simulink model "mg_test18"  (R2017b)
settings: Solver=VariableStepAuto  StartTime=0.0  StopTime=3  MaxStep=1e-4  RelTol=1e-3
values from neighbouring files (symbols this model uses):
  f = 50    [param_mgtest17.m]
  L = 0.15*Pbase/(2*pi*f)    (= 0.000459957785536)    [param_mgtest17.m]
  RL = 1.5e-3*Pbase    (= 0.001445)    [param_mgtest17.m]
  Ts_Power = 1/(fs*100)    (= 2.0202020202e-06)    [param_mgtest17.m]
libraries: powerlib x48, powerlib_meascontrol x15, simulink x8, re_lib x2, electricdrivelib x2, pePowerMeasurement x1
(part 1 of 2)
settings Model: Creator=vijay  LastModifiedBy=btp
settings SFSimCC: SimUseLocalCustomCode=on
settings RTWCC: RTWUseLocalCustomCode=on

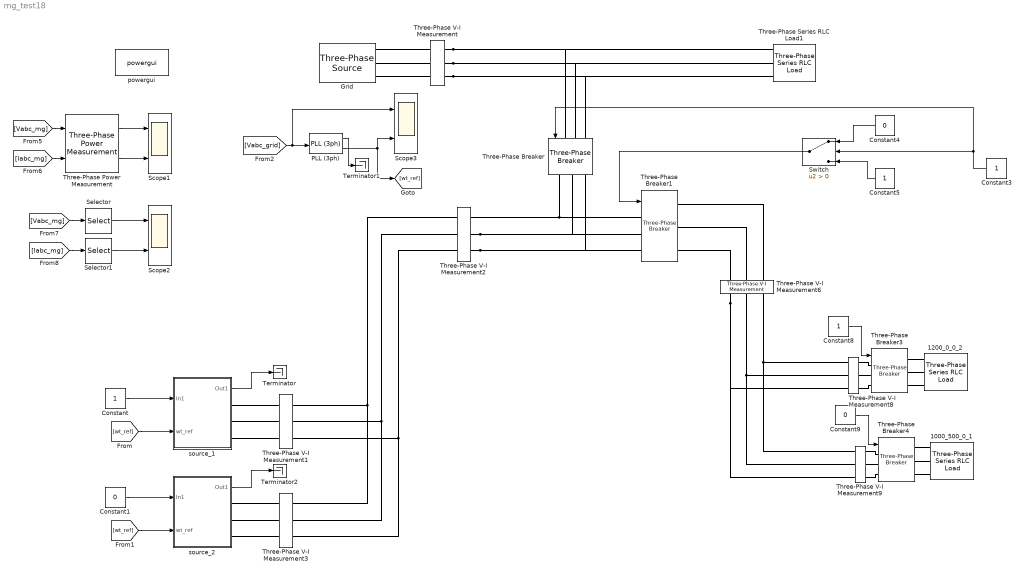
== system mg_test18 ==
  1000_500_0_1 : powerlib/Elements/Three-Phase Series RLC Load  LConnTagsString=A|B|C  Configuration=Y (grounded)  NominalVoltage=230  Vabc=[1e3 1e3 1e3]  Vabcp=[1e3 1e3 1e3]  NominalFrequency=f  UnbalancedPower=off  ActivePower=1e3  InductivePower=500  CapacitivePower=0  Pabc=[10e3 9e3 11e3]  QLabc=[100 90 110]  QCabc=[100 90 110]  Pabcp=[10e3 9e3 11e3]  QLabcp=[100 90 110]  QCabcp=[100 90 110]  Measurements=None  LoadType=constant Z
  1200_0_0_2 : powerlib/Elements/Three-Phase Series RLC Load  LConnTagsString=A|B|C  Configuration=Y (grounded)  NominalVoltage=230  Vabc=[1e3 1e3 1e3]  Vabcp=[1e3 1e3 1e3]  NominalFrequency=f  UnbalancedPower=off  ActivePower=1.2e3  InductivePower=0  CapacitivePower=0  Pabc=[10e3 9e3 11e3]  QLabc=[100 90 110]  QCabc=[100 90 110]  Pabcp=[10e3 9e3 11e3]  QLabcp=[100 90 110]  QCabcp=[100 90 110]  Measurements=None  LoadType=constant Z
  Constant{,3,5,8} (4 alike) : Constant
  Constant1 : Constant  Value=0
  Constant4 : Constant  Value=0
  Constant9 : Constant  Value=0
  Grid : powerlib/Electrical Sources/Three-Phase Source  InternalConnection=Yg  VoltagePhases=off  Voltage=230  PhaseAngle=0  Voltage_phases=[25e3 25e3 25e3]/sqrt(3)  PhaseAngles_phases=[0 -120 +120]  Frequency=f  NonIdealSource=on  SpecifyImpedance=off  Resistance=0.8929  Inductance=16.58e-3  ShortCircuitLevel=100e6  BaseVoltage=230  XRratio=7  BusType=swing  Pref=10e3  Qref=0  Prefabc=[10e3, 10e3, 10e3]  Qrefabc=[0, 0, 0]  Qmin=-inf  Qmax=inf
  PLL (3ph) : powerlib_meascontrol/PLL/PLL (3ph)  Fmin=45  Par_Init=[0, 60]  ParK=[180, 3200, 1]  TcD=1e-4  MaxRateChangeFreq=12  FilterCutOffFreq=25  Ts=0  AGC=on
  Scope1 : Scope  NumInputPorts=2
  Scope2 : Scope  NumInputPorts=2
  Scope3 : Scope  NumInputPorts=2
  Selector : Selector  InputPortWidth=3  IndexOptions=Index vector (dialog)  Indices=[1 ]  OutputSizes=1
  Selector1 : Selector  InputPortWidth=3  IndexOptions=Index vector (dialog)  Indices=[1 ]  OutputSizes=1
  Switch : Switch  Criteria=u2 > Threshold
  Terminator : Terminator
  Terminator1 : Terminator
  Terminator2 : Terminator
  Three-Phase Series RLC Load1 : powerlib/Elements/Three-Phase Series RLC Load  LConnTagsString=A|B|C  Configuration=Y (grounded)  NominalVoltage=230  Vabc=[1e3 1e3 1e3]  Vabcp=[1e3 1e3 1e3]  NominalFrequency=f  UnbalancedPower=off  ActivePower=10e3  InductivePower=0  CapacitivePower=0  Pabc=[10e3 9e3 11e3]  QLabc=[100 90 110]  QCabc=[100 90 110]  Pabcp=[10e3 9e3 11e3]  QLabcp=[100 90 110]  QCabcp=[100 90 110]  Measurements=None  LoadType=constant Z
  Three-Phase V-I Measurement : powerlib/Measurements/Three-Phase V-I Measurement  VoltageMeasurement=phase-to-phase  SetLabelV=on  LabelV=Vabc_grid  Vpu=off  VpuLL=off  CurrentMeasurement=yes  SetLabelI=on  LabelI=Iabc_grid  Ipu=off  Pbase=100e6  Vbase=500e3  OutputType=Complex  PhasorSimulation=off  PSBequivalent=0
  Three-Phase V-I Measurement1 : powerlib/Measurements/Three-Phase V-I Measurement  VoltageMeasurement=phase-to-ground  SetLabelV=on  LabelV=Vabc_s1  Vpu=off  VpuLL=off  CurrentMeasurement=yes  SetLabelI=on  LabelI=Iabc_s1  Ipu=off  Pbase=100e6  Vbase=500e3  OutputType=Complex  PhasorSimulation=off  PSBequivalent=0
  Three-Phase V-I Measurement2 : powerlib/Measurements/Three-Phase V-I Measurement  VoltageMeasurement=phase-to-ground  SetLabelV=on  LabelV=Vabc_mg  Vpu=off  VpuLL=off  CurrentMeasurement=yes  SetLabelI=on  LabelI=Iabc_mg  Ipu=off  Pbase=100e6  Vbase=500e3  OutputType=Complex  PhasorSimulation=off  PSBequivalent=0
  Three-Phase V-I Measurement3 : powerlib/Measurements/Three-Phase V-I Measurement  VoltageMeasurement=phase-to-ground  SetLabelV=on  LabelV=Vabc_s2  Vpu=off  VpuLL=off  CurrentMeasurement=yes  SetLabelI=on  LabelI=Iabc_s2  Ipu=off  Pbase=100e6  Vbase=500e3  OutputType=Complex  PhasorSimulation=off  PSBequivalent=0
  Three-Phase V-I Measurement6 : powerlib/Measurements/Three-Phase V-I Measurement  VoltageMeasurement=phase-to-ground  SetLabelV=on  LabelV=Vabc_mgl  Vpu=off  VpuLL=off  CurrentMeasurement=yes  SetLabelI=on  LabelI=Iabc_mgl  Ipu=off  Pbase=100e6  Vbase=500e3  OutputType=Complex  PhasorSimulation=off  PSBequivalent=0
  Three-Phase V-I Measurement8 : powerlib/Measurements/Three-Phase V-I Measurement  VoltageMeasurement=phase-to-ground  SetLabelV=on  LabelV=Vabc_l2  Vpu=off  VpuLL=off  CurrentMeasurement=yes  SetLabelI=on  LabelI=Iabc_l2  Ipu=off  Pbase=100e6  Vbase=500e3  OutputType=Complex  PhasorSimulation=off  PSBequivalent=0
  Three-Phase V-I Measurement9 : powerlib/Measurements/Three-Phase V-I Measurement  VoltageMeasurement=phase-to-ground  SetLabelV=on  LabelV=Vabc_l3  Vpu=off  VpuLL=off  CurrentMeasurement=yes  SetLabelI=on  LabelI=Iabc_l3  Ipu=off  Pbase=100e6  Vbase=500e3  OutputType=Complex  PhasorSimulation=off  PSBequivalent=0
  Three-Phase Breaker{,1,3..4} (4 alike) : powerlib/Elements/Three-Phase Breaker  InitialState=open  SwitchA=on  SwitchB=on  SwitchC=on  SwitchTimes="[1/60  5/60]"  External=on  BreakerResistance=0.01  SnubberResistance=1e6  SnubberCapacitance=inf  Measurements=None
  Three-Phase Power Measurement : pePowerMeasurement/Three-Phase Power Measurement  OverrideUsingVariant=Continuous  F=f  K=[0 1 2 3]  Seq=Positive  Ts=0
  powergui : powerlib/powergui  Priority=1  SimulationMode=Continuous  SampleTime=Ts_Power  frequency=60  Iterations=50  frequencyindice=0  Pbase=100e6  ErrMax=1e-4  UnitsV=kV  UnitsW=MW  buscounter=0  FunctionMessages=off  echomessages=off  EnableUseOfTLC=off  CurrentSourceSwitches=off  DisableSnubberDevices=off  DisableRonSwitches=off  DisableVfSwitches=off  DisplayEquations=off  SolverType=Tustin/Backward Euler (TBE)  Interpol=off  ExternalGateDelay=off  methode=off  Ts=100  x0status=blocks  SPID=on  SwTol=0  HookPort=off  RestoreLinks=warning  ResistiveCurrentMeasurement=off  Frange=[0:2:500]  Ylog=off  Xlog=on  ShowGrid=off  save=off  variable=ZData  structure=0  ZoomFFT=off  StartTime=0.0  cycles=1  DisplayStyle=1  fundamental=60  FreqAxis=off  MaxFrequency=1000  frequencyindicesteady=1  RmsSteady=1  display=off
  source_1 : Subsystem
  source_2 : Subsystem
  wires:
  source_2/1(Out1) -> Terminator2/1
  [wt_ref] -> source_2/2(wt_ref)
  Constant1/1 -> source_2/1(In1)
  [Vabc_mg] -> Three-Phase Power Measurement/1
  Three-Phase Power Measurement/2 -> Scope1/2
  Three-Phase Power Measurement/1 -> Scope1/1
  [Iabc_mg] -> Three-Phase Power Measurement/2
  Selector1/1 -> Scope2/2
  Selector/1 -> Scope2/1
  Constant8/1 -> Three-Phase Breaker3/1
  [wt_ref] -> source_1/2(wt_ref)
  Constant3/1 -> Three-Phase Breaker/1, Switch/2
  [Vabc_mg] -> Selector/1
  PLL (3ph)/2 -> [wt_ref], Scope3/2
  PLL (3ph)/1 -> Terminator1/1
  Constant/1 -> source_1/1(In1)
  Constant5/1 -> Switch/3
  Switch/1 -> Three-Phase Breaker1/1
  source_1/1(Out1) -> Terminator/1
  [Vabc_grid] -> Scope3/1, PLL (3ph)/1
  Constant4/1 -> Switch/1
  [Iabc_mg] -> Selector1/1
  Constant9/1 -> Three-Phase Breaker4/1
  connections:
  Three-Phase V-I Measurement2/LConn3 -- Three-Phase V-I Measurement3/RConn3 -- Three-Phase V-I Measurement1/RConn3
  Three-Phase V-I Measurement/RConn2 -- Three-Phase Series RLC Load1/LConn2 -- Three-Phase Breaker/LConn2
  Three-Phase V-I Measurement2/LConn1 -- Three-Phase V-I Measurement3/RConn1 -- Three-Phase V-I Measurement1/RConn1
  Three-Phase V-I Measurement2/LConn2 -- Three-Phase V-I Measurement3/RConn2 -- Three-Phase V-I Measurement1/RConn2
  Three-Phase V-I Measurement/RConn3 -- Three-Phase Series RLC Load1/LConn3 -- Three-Phase Breaker/LConn3
  Three-Phase V-I Measurement6/RConn3 -- Three-Phase V-I Measurement9/LConn3 -- Three-Phase V-I Measurement8/LConn3
  Three-Phase V-I Measurement8/LConn2 -- Three-Phase V-I Measurement9/LConn2 -- Three-Phase V-I Measurement6/RConn2
  Three-Phase V-I Measurement2/RConn3 -- Three-Phase Breaker1/LConn3 -- Three-Phase Breaker/RConn3
  Three-Phase V-I Measurement8/LConn1 -- Three-Phase V-I Measurement9/LConn1 -- Three-Phase V-I Measurement6/RConn1
  Three-Phase Breaker1/LConn1 -- Three-Phase Breaker/RConn1 -- Three-Phase V-I Measurement2/RConn1
  Three-Phase V-I Measurement/RConn1 -- Three-Phase Series RLC Load1/LConn1 -- Three-Phase Breaker/LConn1
  Three-Phase V-I Measurement2/RConn2 -- Three-Phase Breaker1/LConn2 -- Three-Phase Breaker/RConn2
  source_2/RConn1 -- Three-Phase V-I Measurement3/LConn1
  Three-Phase Breaker3/RConn2 -- 1200_0_0_2/LConn2
  source_2/RConn2 -- Three-Phase V-I Measurement3/LConn2
  Three-Phase Breaker3/RConn1 -- 1200_0_0_2/LConn1
  source_2/RConn3 -- Three-Phase V-I Measurement3/LConn3
  Three-Phase V-I Measurement8/RConn1 -- Three-Phase Breaker3/LConn1
  Three-Phase V-I Measurement8/RConn3 -- Three-Phase Breaker3/LConn3
  Three-Phase V-I Measurement8/RConn2 -- Three-Phase Breaker3/LConn2
  Grid/RConn2 -- Three-Phase V-I Measurement/LConn2
  Three-Phase V-I Measurement9/RConn1 -- Three-Phase Breaker4/LConn1
  Grid/RConn3 -- Three-Phase V-I Measurement/LConn3
  Three-Phase Breaker4/RConn3 -- 1000_500_0_1/LConn3
  Three-Phase V-I Measurement1/LConn3 -- source_1/RConn3
  Three-Phase V-I Measurement1/LConn1 -- source_1/RConn1
  Grid/RConn1 -- Three-Phase V-I Measurement/LConn1
  Three-Phase V-I Measurement6/LConn2 -- Three-Phase Breaker1/RConn2
  Three-Phase V-I Measurement6/LConn3 -- Three-Phase Breaker1/RConn3
  Three-Phase Breaker4/RConn1 -- 1000_500_0_1/LConn1
  Three-Phase V-I Measurement9/RConn2 -- Three-Phase Breaker4/LConn2
  Three-Phase Breaker3/RConn3 -- 1200_0_0_2/LConn3
  Three-Phase V-I Measurement6/LConn1 -- Three-Phase Breaker1/RConn1
  Three-Phase V-I Measurement9/RConn3 -- Three-Phase Breaker4/LConn3
  Three-Phase V-I Measurement1/LConn2 -- source_1/RConn2
  Three-Phase Breaker4/RConn2 -- 1000_500_0_1/LConn2

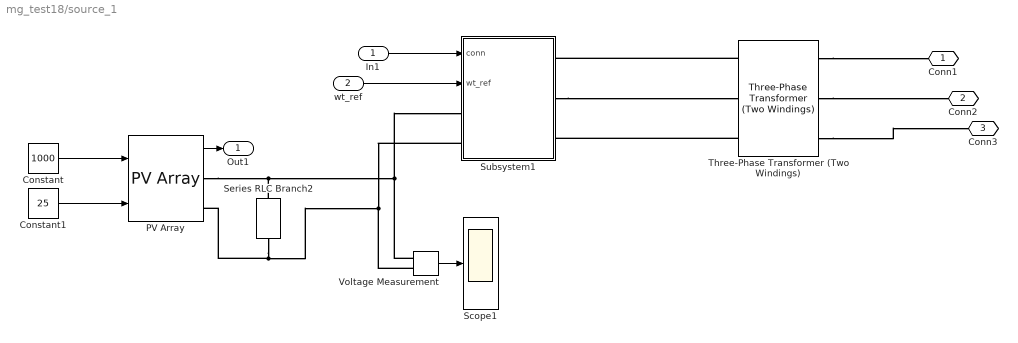
== system mg_test18/source_1 ==
  In1 : Inport
  wt_ref : Inport  Port=2
  Constant : Constant  Value=1000
  Constant1 : Constant  Value=25
  PV Array : re_lib/Solar/PV Array  Npar=6  Nser=2  PlotType=array @ 1000 W/m2 & specified temperatures  S_vec="[ 1000  500  100 ]"  Temp_C_vec="[ 45 25  ]"  ModuleName=Zytech Engineering Technology ZT190S  PlotWhenSelected=off  Pm=190.1592  Ncell=72  Voc=44.86  Isc=5.5  Vm=37.73  Im=5.04  beta_Voc_pc=-0.364  alpha_Isc_pc=0.102  beta_Voc=-0.16329  alpha_Isc=0.00561  IL=5.5086  I0=2.2516e-10  nI=1.0158  Rsh=179.2693  Rs=0.2794  BAL=off  Tc=1e-6  Tfilter=5e-5
  Scope1 : Scope
  Series RLC Branch2 : powerlib/Elements/Series RLC Branch  LConnTagsString=__new0  RConnTagsString=__new0  BranchType=C  Resistance=1  Inductance=100e-3  SetiL0=off  InitialCurrent=0  Capacitance=470e-6  Setx0=on  InitialVoltage=60  Measurements=None
  Subsystem1 : Subsystem
  Three-Phase Transformer (Two Windings) : powerlib/Elements/Three-Phase Transformer (Two Windings)  Winding1Connection=Yg  Winding2Connection=Yg  CoreType=Three single-phase transformers  SetSaturation=off  Hysteresis=off  DataFile='hysteresis'  SetInitialFlux=off  Measurements=None  UNITS=pu  NominalPower=[ 1.2e3 , 50 ]  Winding1=[ 34 , 0.002 , 0.08 ]  Winding2=[ 230 , 0.002 , 0.08 ]  Rm=500  Lm=500  L0=0.5  Saturation=[ 0,0 ; 0.0024,1.2 ; 1.0,1.52 ]  InitialFluxes=[ 0.8 , -0.8 , 0.7 ]  MoreParameters=off  BreakLoop=off  DataType=off  TransfoNumber=1
  Voltage Measurement : powerlib/Measurements/Voltage Measurement  PhasorSimulation=off  OutputType=Complex  PSBequivalent=0
  Conn1 : PMIOPort  Port=1  Side=Right
  Conn2 : PMIOPort  Port=2  Side=Right
  Conn3 : PMIOPort  Port=3  Side=Right
  Out1 : Outport
  wires:
  Constant1/1 -> PV Array/2
  PV Array/1 -> Out1/1
  Constant/1 -> PV Array/1
  Voltage Measurement/1 -> Scope1/1
  In1/1 -> Subsystem1/1(conn)
  wt_ref/1 -> Subsystem1/2(wt_ref)
  connections:
  Subsystem1/RConn2 -- Three-Phase Transformer (Two Windings)/LConn2
  Series RLC Branch2/LConn1 -- Subsystem1/LConn1 -- Voltage Measurement/LConn1 -- PV Array/RConn1
  Three-Phase Transformer (Two Windings)/LConn3 -- Subsystem1/RConn3
  Three-Phase Transformer (Two Windings)/LConn1 -- Subsystem1/RConn1
  Voltage Measurement/LConn2 -- PV Array/RConn2 -- Series RLC Branch2/RConn1 -- Subsystem1/LConn2
  Three-Phase Transformer (Two Windings)/RConn3 -- Conn3/RConn1
  Three-Phase Transformer (Two Windings)/RConn2 -- Conn2/RConn1
  Three-Phase Transformer (Two Windings)/RConn1 -- Conn1/RConn1

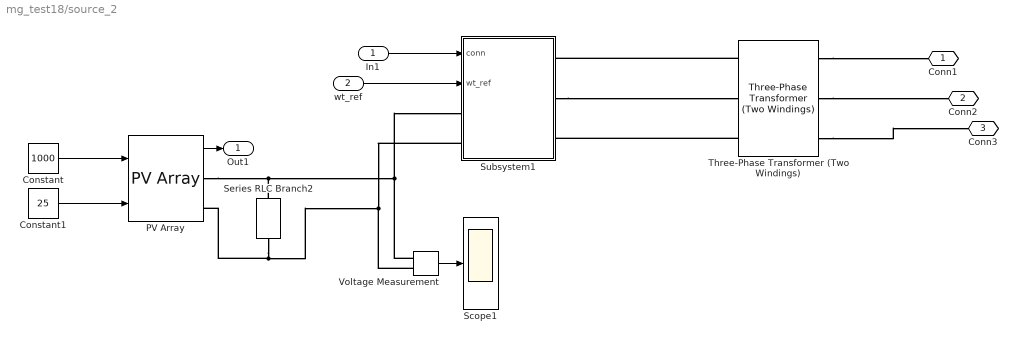
== system mg_test18/source_2 ==
  In1 : Inport
  wt_ref : Inport  Port=2
  Constant : Constant  Value=1000
  Constant1 : Constant  Value=25
  PV Array : re_lib/Solar/PV Array  Npar=6  Nser=2  PlotType=array @ 1000 W/m2 & specified temperatures  S_vec="[ 1000  500  100 ]"  Temp_C_vec="[ 45 25  ]"  ModuleName=Zytech Engineering Technology ZT190S  PlotWhenSelected=off  Pm=190.1592  Ncell=72  Voc=44.86  Isc=5.5  Vm=37.73  Im=5.04  beta_Voc_pc=-0.364  alpha_Isc_pc=0.102  beta_Voc=-0.16329  alpha_Isc=0.00561  IL=5.5086  I0=2.2516e-10  nI=1.0158  Rsh=179.2693  Rs=0.2794  BAL=off  Tc=1e-6  Tfilter=5e-5
  Scope1 : Scope
  Series RLC Branch2 : powerlib/Elements/Series RLC Branch  LConnTagsString=__new0  RConnTagsString=__new0  BranchType=C  Resistance=1  Inductance=100e-3  SetiL0=off  InitialCurrent=0  Capacitance=470e-6  Setx0=on  InitialVoltage=60  Measurements=None
  Subsystem1 : Subsystem
  Three-Phase Transformer (Two Windings) : powerlib/Elements/Three-Phase Transformer (Two Windings)  Winding1Connection=Yg  Winding2Connection=Yg  CoreType=Three single-phase transformers  SetSaturation=off  Hysteresis=off  DataFile='hysteresis'  SetInitialFlux=off  Measurements=None  UNITS=pu  NominalPower=[ 1.2e3 , 50 ]  Winding1=[ 34 , 0.002 , 0.08 ]  Winding2=[ 230 , 0.002 , 0.08 ]  Rm=500  Lm=500  L0=0.5  Saturation=[ 0,0 ; 0.0024,1.2 ; 1.0,1.52 ]  InitialFluxes=[ 0.8 , -0.8 , 0.7 ]  MoreParameters=off  BreakLoop=off  DataType=off  TransfoNumber=1
  Voltage Measurement : powerlib/Measurements/Voltage Measurement  PhasorSimulation=off  OutputType=Complex  PSBequivalent=0
  Conn1 : PMIOPort  Port=1  Side=Right
  Conn2 : PMIOPort  Port=2  Side=Right
  Conn3 : PMIOPort  Port=3  Side=Right
  Out1 : Outport
  wires:
  Constant1/1 -> PV Array/2
  PV Array/1 -> Out1/1
  Constant/1 -> PV Array/1
  Voltage Measurement/1 -> Scope1/1
  In1/1 -> Subsystem1/1(conn)
  wt_ref/1 -> Subsystem1/2(wt_ref)
  connections:
  Subsystem1/RConn2 -- Three-Phase Transformer (Two Windings)/LConn2
  Series RLC Branch2/LConn1 -- Subsystem1/LConn1 -- Voltage Measurement/LConn1 -- PV Array/RConn1
  Three-Phase Transformer (Two Windings)/LConn3 -- Subsystem1/RConn3
  Three-Phase Transformer (Two Windings)/LConn1 -- Subsystem1/RConn1
  Voltage Measurement/LConn2 -- PV Array/RConn2 -- Series RLC Branch2/RConn1 -- Subsystem1/LConn2
  Three-Phase Transformer (Two Windings)/RConn3 -- Conn3/RConn1
  Three-Phase Transformer (Two Windings)/RConn2 -- Conn2/RConn1
  Three-Phase Transformer (Two Windings)/RConn1 -- Conn1/RConn1

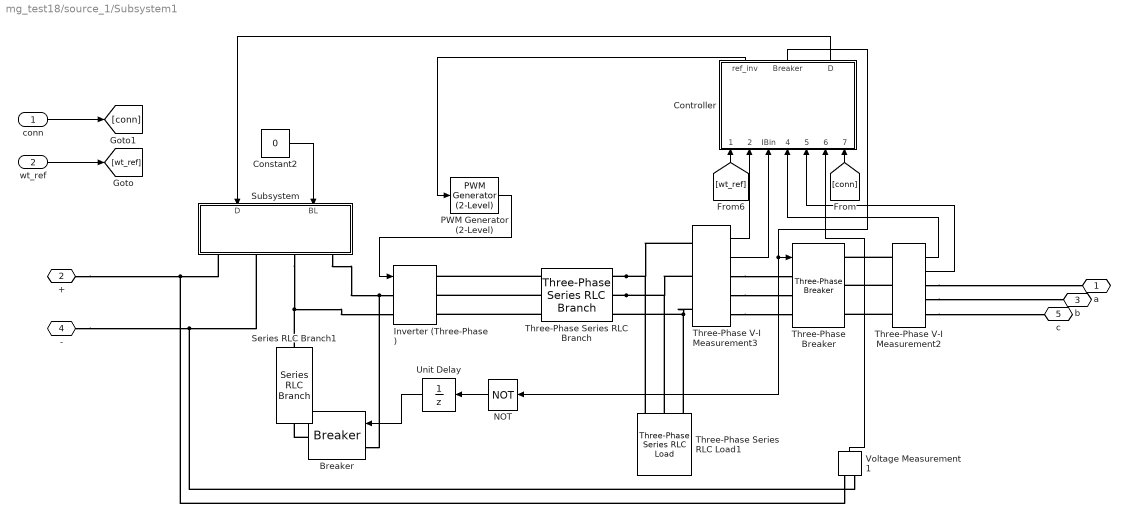
== system mg_test18/source_1/Subsystem1 ==
  conn : Inport
  wt_ref : Inport  Port=2
  Breaker : powerlib/Elements/Breaker  InitialState=0  SwitchingTimes="[1/60  5/60]"  External=on  BreakerResistance=0.01  SnubberResistance=1e6  SnubberCapacitance=inf  Measurements=None  MoreParameters=on  NoBreakLoop=off
      settings: SourceProductName=Simscape Power Systems
  Constant2 : Constant  Value=0
  "Controller " : Subsystem
  Inverter (Three-Phase) : electricdrivelib/Fundamental Drive Blocks/Inverter (Three-Phase)  OverrideUsingVariant=Detailed  detailLevel=Detailed  driveType=Field-oriented control  Ts=2e-6  SnubberResistance=1e6  SnubberCapacitance=inf  Device=IGBT / Diodes  Ron=1e-3  ForwardVoltages=[1.2,1.2]  GTOparameters=[1e-6,2e-6]  IGBTparameters=[1e-6,2e-6]  Measurements=All voltages and currents  converterType=Inverter  SourceFrequency=60  ReferenceFrame=Rotor  dqInductances=[8.5e-3,8.5e-3]  Inductance=8.5e-3  Ls=0  Resistance=0.2  Flux=0.175  Stator_sm=[2.01e-3,4.289e-4,4.477e-3,1.354e-3]  Stator_im=[14.85e-3,0.3027e-3]  Rotor=[9.295e-3,0.3027e-3]  Lm=10.46e-3  p=4
      settings: AttributesFormatString=%<BlockChoice>  SourceProductName=Simscape Power Systems  SourceProductBaseCode=PS
  NOT : Logic  Operator=NOT  IconShape=distinctive  AllPortsSameDT=off  OutDataTypeStr=boolean
  PWM Generator (2-Level) : powerlib_meascontrol/Pulse & Signal Generators/PWM Generator (2-Level)  ModulatorType=Three-phase bridge (6 pulses)  ModulatorMode=Unsynchronized  Fc=fs  Pc=90  nF=27  MinMax="[ -1  1 ]"  SamplingTechnique=Natural  ModulatingSignals=off  m=0.8  Freq=60  Phase=0  Ts=Ts_Power  ShowCarrierOutport=off
      settings: SourceProductName=Simscape Power Systems
  Series RLC Branch1 : powerlib/Elements/Series RLC Branch  LConnTagsString=__new0  RConnTagsString=__new0  BranchType=R  Resistance=1.92  Inductance=1e-3  SetiL0=off  InitialCurrent=0  Capacitance=1e-6  Setx0=off  InitialVoltage=0  Measurements=None
  Subsystem : Subsystem
  Three-Phase Series RLC Branch : powerlib/Elements/Three-Phase Series RLC Branch  LConnTagsString=A|B|C  RConnTagsString=A|B|C  BranchType=RL  Resistance=RL  Inductance=L  Capacitance=1e-6  Measurements=None
  Three-Phase Series RLC Load1 : powerlib/Elements/Three-Phase Series RLC Load  LConnTagsString=A|B|C  Configuration=Delta  NominalVoltage=Vbase  Vabc=[1e3 1e3 1e3]  Vabcp=[1e3 1e3 1e3]  NominalFrequency=f  UnbalancedPower=off  ActivePower=Pc  InductivePower=0  CapacitivePower=Qc  Pabc=[10e3 9e3 11e3]  QLabc=[100 90 110]  QCabc=[100 90 110]  Pabcp=[10e3 9e3 11e3]  QLabcp=[100 90 110]  QCabcp=[100 90 110]  Measurements=None  LoadType=constant Z
  Three-Phase V-I Measurement2 : powerlib/Measurements/Three-Phase V-I Measurement  VoltageMeasurement=phase-to-phase  SetLabelV=off  LabelV=v2  Vpu=off  VpuLL=off  CurrentMeasurement=yes  SetLabelI=off  LabelI=i2  Ipu=off  Pbase=100e6  Vbase=500e3  OutputType=Complex  PhasorSimulation=off  PSBequivalent=0
  Three-Phase V-I Measurement3 : powerlib/Measurements/Three-Phase V-I Measurement  VoltageMeasurement=phase-to-phase  SetLabelV=off  LabelV=v1  Vpu=off  VpuLL=off  CurrentMeasurement=yes  SetLabelI=off  LabelI=i1  Ipu=off  Pbase=100e6  Vbase=500e3  OutputType=Complex  PhasorSimulation=off  PSBequivalent=0
  Three-Phase Breaker : powerlib/Elements/Three-Phase Breaker  InitialState=open  SwitchA=on  SwitchB=on  SwitchC=on  SwitchTimes="[1/60  5/60]"  External=on  BreakerResistance=0.01  SnubberResistance=1e6  SnubberCapacitance=inf  Measurements=None
  Unit Delay : UnitDelay  InitialCondition=1  SampleTime=-1
  Voltage Measurement1 : powerlib/Measurements/Voltage Measurement  PhasorSimulation=off  OutputType=Complex  PSBequivalent=0
  a : PMIOPort  Port=1  Side=Right
  + : PMIOPort  Port=2  Side=Left
  b : PMIOPort  Port=3  Side=Right
  - : PMIOPort  Port=4  Side=Left
  c : PMIOPort  Port=5  Side=Right
  wires:
  PWM Generator (2-Level)/1 -> Inverter (Three-Phase)/1
  Constant2/1 -> Subsystem/2(BL)
  wt_ref/1 -> [wt_ref]
  conn/1 -> [conn]
  Three-Phase V-I Measurement3/1 -> "Controller "/2("VBin ")
  Three-Phase V-I Measurement3/2 -> "Controller "/3(IBin)
  Three-Phase V-I Measurement2/1 -> "Controller "/4(VBout)
  Three-Phase V-I Measurement2/2 -> "Controller "/5(IBout)
  Voltage Measurement1/1 -> "Controller "/6(In_DC)
  [conn] -> "Controller "/7(connect_o)
  [wt_ref] -> "Controller "/1(wt_ref)
  "Controller "/1(ref_inv) -> PWM Generator (2-Level)/1
  "Controller "/2("Breaker ") -> NOT/1, Three-Phase Breaker/1
  "Controller "/3("D ") -> Subsystem/1(D)
  NOT/1 -> Unit Delay/1
  Unit Delay/1 -> Breaker/1
  connections:
  Three-Phase V-I Measurement2/LConn2 -- Three-Phase Breaker/RConn2
  Voltage Measurement1/LConn1 -- +/RConn1 -- Subsystem/RConn1
  Voltage Measurement1/LConn2 -- Subsystem/RConn2 -- -/RConn1
  Three-Phase V-I Measurement3/RConn1 -- Three-Phase Breaker/LConn1
  Three-Phase V-I Measurement3/RConn3 -- Three-Phase Breaker/LConn3
  Subsystem/RConn4 -- Breaker/LConn1 -- Inverter (Three-Phase)/LConn1
  Three-Phase V-I Measurement2/LConn1 -- Three-Phase Breaker/RConn1
  Three-Phase V-I Measurement2/LConn3 -- Three-Phase Breaker/RConn3
  Subsystem/RConn3 -- Series RLC Branch1/LConn1 -- Inverter (Three-Phase)/LConn2
  Three-Phase V-I Measurement3/RConn2 -- Three-Phase Breaker/LConn2
  Three-Phase V-I Measurement2/RConn1 -- a/RConn1
  Three-Phase V-I Measurement2/RConn3 -- c/RConn1
  Three-Phase V-I Measurement2/RConn2 -- b/RConn1
  Three-Phase V-I Measurement3/LConn3 -- Three-Phase Series RLC Branch/RConn3 -- Three-Phase Series RLC Load1/LConn3
  Three-Phase Series RLC Branch/RConn1 -- Three-Phase V-I Measurement3/LConn1 -- Three-Phase Series RLC Load1/LConn1
  Three-Phase Series RLC Branch/RConn2 -- Three-Phase V-I Measurement3/LConn2 -- Three-Phase Series RLC Load1/LConn2
  Three-Phase Series RLC Branch/LConn3 -- Inverter (Three-Phase)/RConn3
  Three-Phase Series RLC Branch/LConn2 -- Inverter (Three-Phase)/RConn2
  Three-Phase Series RLC Branch/LConn1 -- Inverter (Three-Phase)/RConn1
  Breaker/RConn1 -- Series RLC Branch1/RConn1

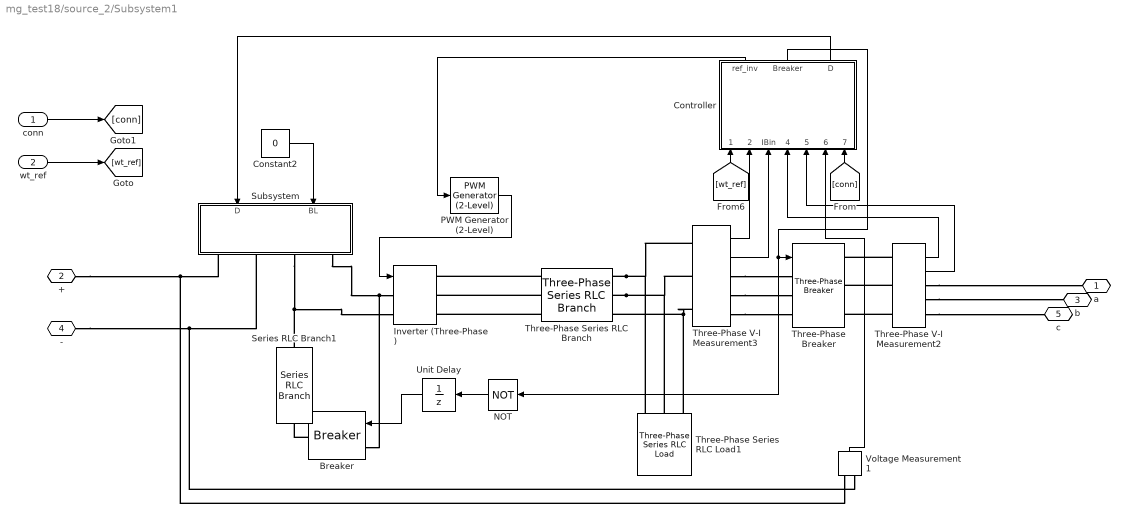
== system mg_test18/source_2/Subsystem1 ==
  conn : Inport
  wt_ref : Inport  Port=2
  Breaker : powerlib/Elements/Breaker  InitialState=0  SwitchingTimes="[1/60  5/60]"  External=on  BreakerResistance=0.01  SnubberResistance=1e6  SnubberCapacitance=inf  Measurements=None  MoreParameters=on  NoBreakLoop=off
      settings: SourceProductName=Simscape Power Systems
  Constant2 : Constant  Value=0
  "Controller " : Subsystem
  Inverter (Three-Phase) : electricdrivelib/Fundamental Drive Blocks/Inverter (Three-Phase)  OverrideUsingVariant=Detailed  detailLevel=Detailed  driveType=Field-oriented control  Ts=2e-6  SnubberResistance=1e6  SnubberCapacitance=inf  Device=IGBT / Diodes  Ron=1e-3  ForwardVoltages=[1.2,1.2]  GTOparameters=[1e-6,2e-6]  IGBTparameters=[1e-6,2e-6]  Measurements=All voltages and currents  converterType=Inverter  SourceFrequency=60  ReferenceFrame=Rotor  dqInductances=[8.5e-3,8.5e-3]  Inductance=8.5e-3  Ls=0  Resistance=0.2  Flux=0.175  Stator_sm=[2.01e-3,4.289e-4,4.477e-3,1.354e-3]  Stator_im=[14.85e-3,0.3027e-3]  Rotor=[9.295e-3,0.3027e-3]  Lm=10.46e-3  p=4
      settings: AttributesFormatString=%<BlockChoice>  SourceProductName=Simscape Power Systems  SourceProductBaseCode=PS
  NOT : Logic  Operator=NOT  IconShape=distinctive  AllPortsSameDT=off  OutDataTypeStr=boolean
  PWM Generator (2-Level) : powerlib_meascontrol/Pulse & Signal Generators/PWM Generator (2-Level)  ModulatorType=Three-phase bridge (6 pulses)  ModulatorMode=Unsynchronized  Fc=fs  Pc=90  nF=27  MinMax="[ -1  1 ]"  SamplingTechnique=Natural  ModulatingSignals=off  m=0.8  Freq=60  Phase=0  Ts=Ts_Power  ShowCarrierOutport=off
      settings: SourceProductName=Simscape Power Systems
  Series RLC Branch1 : powerlib/Elements/Series RLC Branch  LConnTagsString=__new0  RConnTagsString=__new0  BranchType=R  Resistance=1.92  Inductance=1e-3  SetiL0=off  InitialCurrent=0  Capacitance=1e-6  Setx0=off  InitialVoltage=0  Measurements=None
  Subsystem : Subsystem
  Three-Phase Series RLC Branch : powerlib/Elements/Three-Phase Series RLC Branch  LConnTagsString=A|B|C  RConnTagsString=A|B|C  BranchType=RL  Resistance=RL  Inductance=L  Capacitance=1e-6  Measurements=None
  Three-Phase Series RLC Load1 : powerlib/Elements/Three-Phase Series RLC Load  LConnTagsString=A|B|C  Configuration=Delta  NominalVoltage=Vbase  Vabc=[1e3 1e3 1e3]  Vabcp=[1e3 1e3 1e3]  NominalFrequency=f  UnbalancedPower=off  ActivePower=Pc  InductivePower=0  CapacitivePower=Qc  Pabc=[10e3 9e3 11e3]  QLabc=[100 90 110]  QCabc=[100 90 110]  Pabcp=[10e3 9e3 11e3]  QLabcp=[100 90 110]  QCabcp=[100 90 110]  Measurements=None  LoadType=constant Z
  Three-Phase V-I Measurement2 : powerlib/Measurements/Three-Phase V-I Measurement  VoltageMeasurement=phase-to-phase  SetLabelV=off  LabelV=v2  Vpu=off  VpuLL=off  CurrentMeasurement=yes  SetLabelI=off  LabelI=i2  Ipu=off  Pbase=100e6  Vbase=500e3  OutputType=Complex  PhasorSimulation=off  PSBequivalent=0
  Three-Phase V-I Measurement3 : powerlib/Measurements/Three-Phase V-I Measurement  VoltageMeasurement=phase-to-phase  SetLabelV=off  LabelV=v1  Vpu=off  VpuLL=off  CurrentMeasurement=yes  SetLabelI=off  LabelI=i1  Ipu=off  Pbase=100e6  Vbase=500e3  OutputType=Complex  PhasorSimulation=off  PSBequivalent=0
  Three-Phase Breaker : powerlib/Elements/Three-Phase Breaker  InitialState=open  SwitchA=on  SwitchB=on  SwitchC=on  SwitchTimes="[1/60  5/60]"  External=on  BreakerResistance=0.01  SnubberResistance=1e6  SnubberCapacitance=inf  Measurements=None
  Unit Delay : UnitDelay  InitialCondition=1  SampleTime=-1
  Voltage Measurement1 : powerlib/Measurements/Voltage Measurement  PhasorSimulation=off  OutputType=Complex  PSBequivalent=0
  a : PMIOPort  Port=1  Side=Right
  + : PMIOPort  Port=2  Side=Left
  b : PMIOPort  Port=3  Side=Right
  - : PMIOPort  Port=4  Side=Left
  c : PMIOPort  Port=5  Side=Right
  wires:
  PWM Generator (2-Level)/1 -> Inverter (Three-Phase)/1
  Constant2/1 -> Subsystem/2(BL)
  wt_ref/1 -> [wt_ref]
  conn/1 -> [conn]
  Three-Phase V-I Measurement3/1 -> "Controller "/2("VBin ")
  Three-Phase V-I Measurement3/2 -> "Controller "/3(IBin)
  Three-Phase V-I Measurement2/1 -> "Controller "/4(VBout)
  Three-Phase V-I Measurement2/2 -> "Controller "/5(IBout)
  Voltage Measurement1/1 -> "Controller "/6(In_DC)
  [conn] -> "Controller "/7(connect_o)
  [wt_ref] -> "Controller "/1(wt_ref)
  "Controller "/1(ref_inv) -> PWM Generator (2-Level)/1
  "Controller "/2("Breaker ") -> NOT/1, Three-Phase Breaker/1
  "Controller "/3("D ") -> Subsystem/1(D)
  NOT/1 -> Unit Delay/1
  Unit Delay/1 -> Breaker/1
  connections:
  Three-Phase V-I Measurement2/LConn2 -- Three-Phase Breaker/RConn2
  Voltage Measurement1/LConn1 -- +/RConn1 -- Subsystem/RConn1
  Voltage Measurement1/LConn2 -- Subsystem/RConn2 -- -/RConn1
  Three-Phase V-I Measurement3/RConn1 -- Three-Phase Breaker/LConn1
  Three-Phase V-I Measurement3/RConn3 -- Three-Phase Breaker/LConn3
  Subsystem/RConn4 -- Inverter (Three-Phase)/LConn1 -- Breaker/LConn1
  Three-Phase V-I Measurement2/LConn1 -- Three-Phase Breaker/RConn1
  Three-Phase V-I Measurement2/LConn3 -- Three-Phase Breaker/RConn3
  Subsystem/RConn3 -- Inverter (Three-Phase)/LConn2 -- Series RLC Branch1/LConn1
  Three-Phase V-I Measurement3/RConn2 -- Three-Phase Breaker/LConn2
  Three-Phase V-I Measurement2/RConn1 -- a/RConn1
  Three-Phase V-I Measurement2/RConn3 -- c/RConn1
  Three-Phase V-I Measurement2/RConn2 -- b/RConn1
  Three-Phase V-I Measurement3/LConn3 -- Three-Phase Series RLC Branch/RConn3 -- Three-Phase Series RLC Load1/LConn3
  Three-Phase Series RLC Branch/RConn1 -- Three-Phase V-I Measurement3/LConn1 -- Three-Phase Series RLC Load1/LConn1
  Three-Phase Series RLC Branch/RConn2 -- Three-Phase V-I Measurement3/LConn2 -- Three-Phase Series RLC Load1/LConn2
  Three-Phase Series RLC Branch/LConn3 -- Inverter (Three-Phase)/RConn3
  Three-Phase Series RLC Branch/LConn2 -- Inverter (Three-Phase)/RConn2
  Three-Phase Series RLC Branch/LConn1 -- Inverter (Three-Phase)/RConn1
  Breaker/RConn1 -- Series RLC Branch1/RConn1

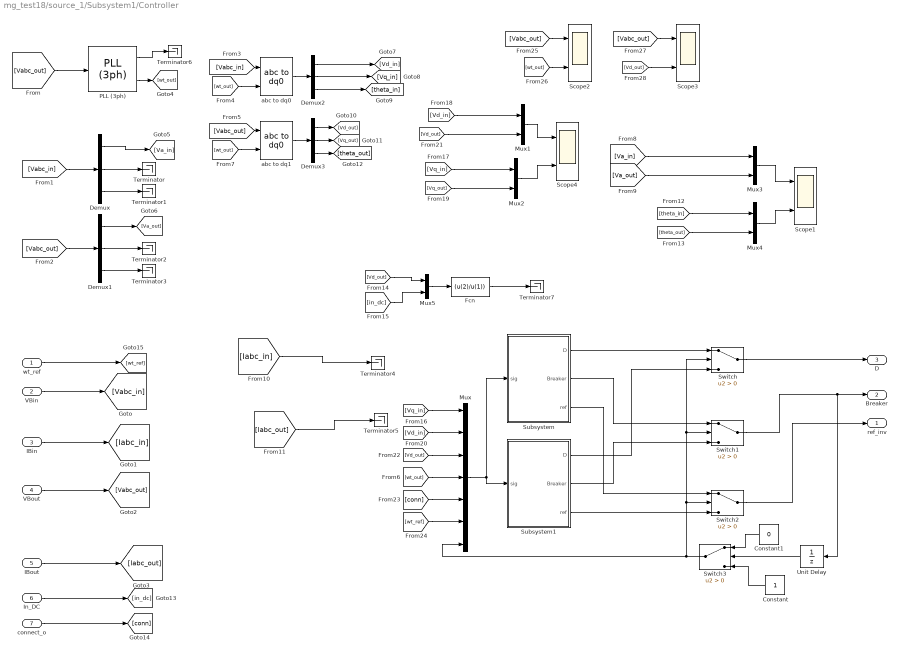
== system mg_test18/source_1/Subsystem1/Controller  ==
  wt_ref : Inport
  "VBin " : Inport  Port=2
  IBin : Inport  Port=3
  VBout : Inport  Port=4
  IBout : Inport  Port=5
  In_DC : Inport  Port=6
  connect_o : Inport  Port=7
  Constant : Constant
  Constant1 : Constant  Value=0
  Demux{,1..3} (4 alike) : Demux  Outputs=3
  Fcn : Fcn  Expr=(u(2)/u(1))
  Mux : Mux  Inputs=7
  Mux{1..5} (5 alike) : Mux  Inputs=2
  PLL (3ph) : powerlib_meascontrol/PLL/PLL (3ph)  Fmin=45  Par_Init=[0, f]  ParK=[180, 3200, 1]  TcD=1e-4  MaxRateChangeFreq=12  FilterCutOffFreq=25  Ts=Ts_Power  AGC=on
  Scope{1..4} (4 alike) : Scope  NumInputPorts=2
  Subsystem : Subsystem
  Subsystem1 : Subsystem
  Switch{,1..3} (4 alike) : Switch  Criteria=u2 > Threshold
  Terminator{,1..7} (8 alike) : Terminator
  Unit Delay : UnitDelay  SampleTime=Ts_Power
  abc to dq0 : powerlib_meascontrol/Transformations/abc to dq0  Alignment=90 degrees behind phase A axis
  abc to dq1 : powerlib_meascontrol/Transformations/abc to dq0  Alignment=90 degrees behind phase A axis
  ref_inv : Outport
  "Breaker " : Outport  Port=2
  "D " : Outport  Port=3
  wires:
  [Vd_out] -> Scope3/2
  [Vq_out] -> Mux2/2
  [wt_ref] -> Mux/6
  abc to dq1/1 -> Demux3/1
  [wt_out] -> Scope2/2
  [Vabc_out] -> Scope2/1
  [Iabc_out] -> Terminator5/1
  "VBin "/1 -> [Vabc_in]
  abc to dq0/1 -> Demux2/1
  Subsystem1/1(D) -> Switch/3
  [Vq_in] -> Mux/1
  Subsystem/2(Breaker) -> Switch1/1
  [Vq_in] -> Mux2/1
  [wt_out] -> abc to dq1/2
  PLL (3ph)/1 -> Terminator6/1
  In_DC/1 -> [in_dc]
  Switch1/1 -> Unit Delay/1, "Breaker "/1
  [conn] -> Mux/5
  Demux3/2 -> [Vq_out]
  [Vd_in] -> Mux/2
  Demux/2 -> Terminator/1
  Mux5/1 -> Fcn/1
  Switch2/1 -> ref_inv/1
  Fcn/1 -> Terminator7/1
  Subsystem/1(D) -> Switch/1
  [wt_out] -> Mux/4
  [Vd_out] -> Mux5/1
  Switch/1 -> "D "/1
  Mux/1 -> Subsystem/1(sig), Subsystem1/1(sig)
  [wt_out] -> abc to dq0/2
  [in_dc] -> Mux5/2
  [theta_out] -> Mux4/2
  [Vd_in] -> Mux1/1
  Mux2/1 -> Scope4/2
  [theta_in] -> Mux4/1
  wt_ref/1 -> [wt_ref]
  Mux4/1 -> Scope1/2
  Demux3/1 -> [Vd_out]
  Demux/1 -> [Va_in]
  connect_o/1 -> [conn]
  Mux1/1 -> Scope4/1
  Subsystem1/2(Breaker) -> Switch1/3
  [Vabc_in] -> abc to dq0/1
  [Vd_out] -> Mux1/2
  Subsystem/3(ref) -> Switch2/1
  Demux1/3 -> Terminator3/1
  [Va_in] -> Mux3/1
  Demux1/2 -> Terminator2/1
  [Iabc_in] -> Terminator4/1
  Demux/3 -> Terminator1/1
  [Vabc_out] -> PLL (3ph)/1
  [Vd_out] -> Mux/3
  [Vabc_out] -> abc to dq1/1
  [Va_out] -> Mux3/2
  Mux3/1 -> Scope1/1
  VBout/1 -> [Vabc_out]
  [Vabc_out] -> Demux1/1
  [Vabc_in] -> Demux/1
  PLL (3ph)/2 -> [wt_out]
  Subsystem1/3(ref) -> Switch2/3
  IBout/1 -> [Iabc_out]
  [Vabc_out] -> Scope3/1
  Demux3/3 -> [theta_out]
  IBin/1 -> [Iabc_in]
  Demux1/1 -> [Va_out]
  Demux2/3 -> [theta_in]
  Demux2/2 -> [Vq_in]
  Demux2/1 -> [Vd_in]
  Switch3/1 -> Switch/2, Switch1/2, Switch2/2, Mux/7
  Unit Delay/1 -> Switch3/2
  Constant/1 -> Switch3/3
  Constant1/1 -> Switch3/1

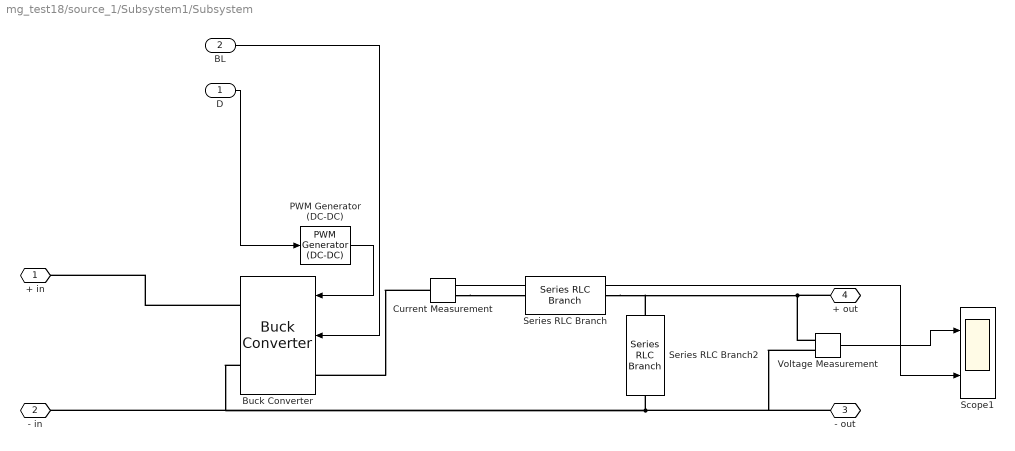
== system mg_test18/source_1/Subsystem1/Subsystem ==
  D : Inport
  BL : Inport  Port=2
  Buck Converter : powerlib/Power Electronics/Buck Converter  ModelType=Switching devices  Ron=1e-3  Rs=1e6  Cs=inf  Vforward=[0,0]  Ron_Diode=1e-3  Rs_Diode=1e6  Cs_Diode=inf  Vf_Diode=1e-3  Rs_CurrentSource=inf
      settings: SourceProductName=Simscape Power Systems  SourceProductBaseCode=PS
  Current Measurement : powerlib/Measurements/Current Measurement  PhasorSimulation=off  OutputType=Complex  PSBequivalent=0
  PWM Generator (DC-DC) : powerlib_meascontrol/Pulse & Signal Generators/PWM Generator (DC-DC)  Fsw=20000  Ts=0
  Scope1 : Scope  NumInputPorts=2
  Series RLC Branch : powerlib/Elements/Series RLC Branch  LConnTagsString=__new0  RConnTagsString=__new0  BranchType=L  Resistance=1  Inductance=96e-6  SetiL0=off  InitialCurrent=0  Capacitance=1e-6  Setx0=off  InitialVoltage=0  Measurements=None
  Series RLC Branch2 : powerlib/Elements/Series RLC Branch  LConnTagsString=__new0  RConnTagsString=__new0  BranchType=C  Resistance=1  Inductance=100e-3  SetiL0=off  InitialCurrent=0  Capacitance=470e-6  Setx0=on  InitialVoltage=0  Measurements=None
  Voltage Measurement : powerlib/Measurements/Voltage Measurement  PhasorSimulation=off  OutputType=Complex  PSBequivalent=0
  + in : PMIOPort  Port=1  Side=Right
  "- in " : PMIOPort  Port=2  Side=Right
  - out : PMIOPort  Port=3  Side=Right
  "+ out " : PMIOPort  Port=4  Side=Right
  wires:
  PWM Generator (DC-DC)/1 -> Buck Converter/1
  D/1 -> PWM Generator (DC-DC)/1
  Voltage Measurement/1 -> Scope1/1
  Current Measurement/1 -> Scope1/2
  BL/1 -> Buck Converter/2
  connections:
  Voltage Measurement/LConn1 -- Series RLC Branch/RConn1 -- Series RLC Branch2/LConn1 -- "+ out "/RConn1
  Series RLC Branch2/RConn1 -- - out/RConn1 -- Voltage Measurement/LConn2 -- "- in "/RConn1 -- Buck Converter/RConn2
  Current Measurement/RConn1 -- Series RLC Branch/LConn1
  Current Measurement/LConn1 -- Buck Converter/LConn1
  Buck Converter/RConn1 -- + in/RConn1

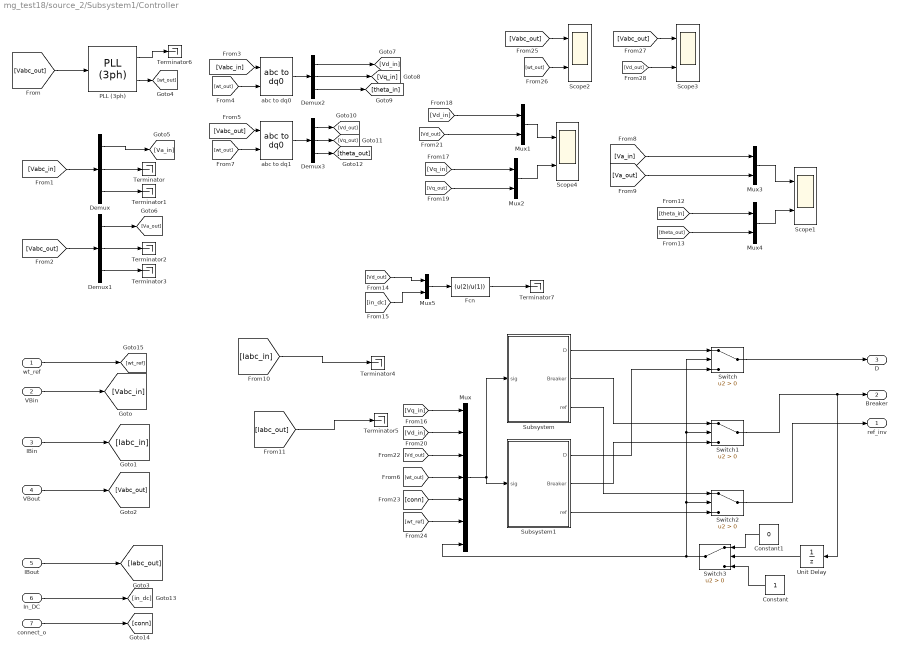
== system mg_test18/source_2/Subsystem1/Controller  ==
  wt_ref : Inport
  "VBin " : Inport  Port=2
  IBin : Inport  Port=3
  VBout : Inport  Port=4
  IBout : Inport  Port=5
  In_DC : Inport  Port=6
  connect_o : Inport  Port=7
  Constant : Constant
  Constant1 : Constant  Value=0
  Demux{,1..3} (4 alike) : Demux  Outputs=3
  Fcn : Fcn  Expr=(u(2)/u(1))
  Mux : Mux  Inputs=7
  Mux{1..5} (5 alike) : Mux  Inputs=2
  PLL (3ph) : powerlib_meascontrol/PLL/PLL (3ph)  Fmin=45  Par_Init=[0, f]  ParK=[180, 3200, 1]  TcD=1e-4  MaxRateChangeFreq=12  FilterCutOffFreq=25  Ts=Ts_Power  AGC=on
  Scope{1..4} (4 alike) : Scope  NumInputPorts=2
  Subsystem : Subsystem
  Subsystem1 : Subsystem
  Switch{,1..3} (4 alike) : Switch  Criteria=u2 > Threshold
  Terminator{,1..7} (8 alike) : Terminator
  Unit Delay : UnitDelay  SampleTime=Ts_Power
  abc to dq0 : powerlib_meascontrol/Transformations/abc to dq0  Alignment=90 degrees behind phase A axis
  abc to dq1 : powerlib_meascontrol/Transformations/abc to dq0  Alignment=90 degrees behind phase A axis
  ref_inv : Outport
  "Breaker " : Outport  Port=2
  "D " : Outport  Port=3
  wires:
  [Vd_out] -> Scope3/2
  [Vq_out] -> Mux2/2
  [wt_ref] -> Mux/6
  abc to dq1/1 -> Demux3/1
  [wt_out] -> Scope2/2
  [Vabc_out] -> Scope2/1
  [Iabc_out] -> Terminator5/1
  "VBin "/1 -> [Vabc_in]
  abc to dq0/1 -> Demux2/1
  Subsystem1/1(D) -> Switch/3
  [Vq_in] -> Mux/1
  Subsystem/2(Breaker) -> Switch1/1
  [Vq_in] -> Mux2/1
  [wt_out] -> abc to dq1/2
  PLL (3ph)/1 -> Terminator6/1
  In_DC/1 -> [in_dc]
  Switch1/1 -> Unit Delay/1, "Breaker "/1
  [conn] -> Mux/5
  Demux3/2 -> [Vq_out]
  [Vd_in] -> Mux/2
  Demux/2 -> Terminator/1
  Mux5/1 -> Fcn/1
  Switch2/1 -> ref_inv/1
  Fcn/1 -> Terminator7/1
  Subsystem/1(D) -> Switch/1
  [wt_out] -> Mux/4
  [Vd_out] -> Mux5/1
  Switch/1 -> "D "/1
  Mux/1 -> Subsystem/1(sig), Subsystem1/1(sig)
  [wt_out] -> abc to dq0/2
  [in_dc] -> Mux5/2
  [theta_out] -> Mux4/2
  [Vd_in] -> Mux1/1
  Mux2/1 -> Scope4/2
  [theta_in] -> Mux4/1
  wt_ref/1 -> [wt_ref]
  Mux4/1 -> Scope1/2
  Demux3/1 -> [Vd_out]
  Demux/1 -> [Va_in]
  connect_o/1 -> [conn]
  Mux1/1 -> Scope4/1
  Subsystem1/2(Breaker) -> Switch1/3
  [Vabc_in] -> abc to dq0/1
  [Vd_out] -> Mux1/2
  Subsystem/3(ref) -> Switch2/1
  Demux1/3 -> Terminator3/1
  [Va_in] -> Mux3/1
  Demux1/2 -> Terminator2/1
  [Iabc_in] -> Terminator4/1
  Demux/3 -> Terminator1/1
  [Vabc_out] -> PLL (3ph)/1
  [Vd_out] -> Mux/3
  [Vabc_out] -> abc to dq1/1
  [Va_out] -> Mux3/2
  Mux3/1 -> Scope1/1
  VBout/1 -> [Vabc_out]
  [Vabc_out] -> Demux1/1
  [Vabc_in] -> Demux/1
  PLL (3ph)/2 -> [wt_out]
  Subsystem1/3(ref) -> Switch2/3
  IBout/1 -> [Iabc_out]
  [Vabc_out] -> Scope3/1
  Demux3/3 -> [theta_out]
  IBin/1 -> [Iabc_in]
  Demux1/1 -> [Va_out]
  Demux2/3 -> [theta_in]
  Demux2/2 -> [Vq_in]
  Demux2/1 -> [Vd_in]
  Switch3/1 -> Switch/2, Switch1/2, Switch2/2, Mux/7
  Unit Delay/1 -> Switch3/2
  Constant/1 -> Switch3/3
  Constant1/1 -> Switch3/1

== system mg_test18/source_2/Subsystem1/Subsystem ==
  D : Inport
  BL : Inport  Port=2
  Buck Converter : powerlib/Power Electronics/Buck Converter  ModelType=Switching devices  Ron=1e-3  Rs=1e6  Cs=inf  Vforward=[0,0]  Ron_Diode=1e-3  Rs_Diode=1e6  Cs_Diode=inf  Vf_Diode=1e-3  Rs_CurrentSource=inf
      settings: SourceProductName=Simscape Power Systems  SourceProductBaseCode=PS
  Current Measurement : powerlib/Measurements/Current Measurement  PhasorSimulation=off  OutputType=Complex  PSBequivalent=0
  PWM Generator (DC-DC) : powerlib_meascontrol/Pulse & Signal Generators/PWM Generator (DC-DC)  Fsw=20000  Ts=0
  Scope1 : Scope  NumInputPorts=2
  Series RLC Branch : powerlib/Elements/Series RLC Branch  LConnTagsString=__new0  RConnTagsString=__new0  BranchType=L  Resistance=1  Inductance=96e-6  SetiL0=off  InitialCurrent=0  Capacitance=1e-6  Setx0=off  InitialVoltage=0  Measurements=None
  Series RLC Branch2 : powerlib/Elements/Series RLC Branch  LConnTagsString=__new0  RConnTagsString=__new0  BranchType=C  Resistance=1  Inductance=100e-3  SetiL0=off  InitialCurrent=0  Capacitance=470e-6  Setx0=on  InitialVoltage=0  Measurements=None
  Voltage Measurement : powerlib/Measurements/Voltage Measurement  PhasorSimulation=off  OutputType=Complex  PSBequivalent=0
  + in : PMIOPort  Port=1  Side=Right
  "- in " : PMIOPort  Port=2  Side=Right
  - out : PMIOPort  Port=3  Side=Right
  "+ out " : PMIOPort  Port=4  Side=Right
  wires:
  PWM Generator (DC-DC)/1 -> Buck Converter/1
  D/1 -> PWM Generator (DC-DC)/1
  Voltage Measurement/1 -> Scope1/1
  Current Measurement/1 -> Scope1/2
  BL/1 -> Buck Converter/2
  connections:
  Voltage Measurement/LConn1 -- "+ out "/RConn1 -- Series RLC Branch/RConn1 -- Series RLC Branch2/LConn1
  Series RLC Branch2/RConn1 -- "- in "/RConn1 -- Buck Converter/RConn2 -- - out/RConn1 -- Voltage Measurement/LConn2
  Current Measurement/RConn1 -- Series RLC Branch/LConn1
  Current Measurement/LConn1 -- Buck Converter/LConn1
  Buck Converter/RConn1 -- + in/RConn1

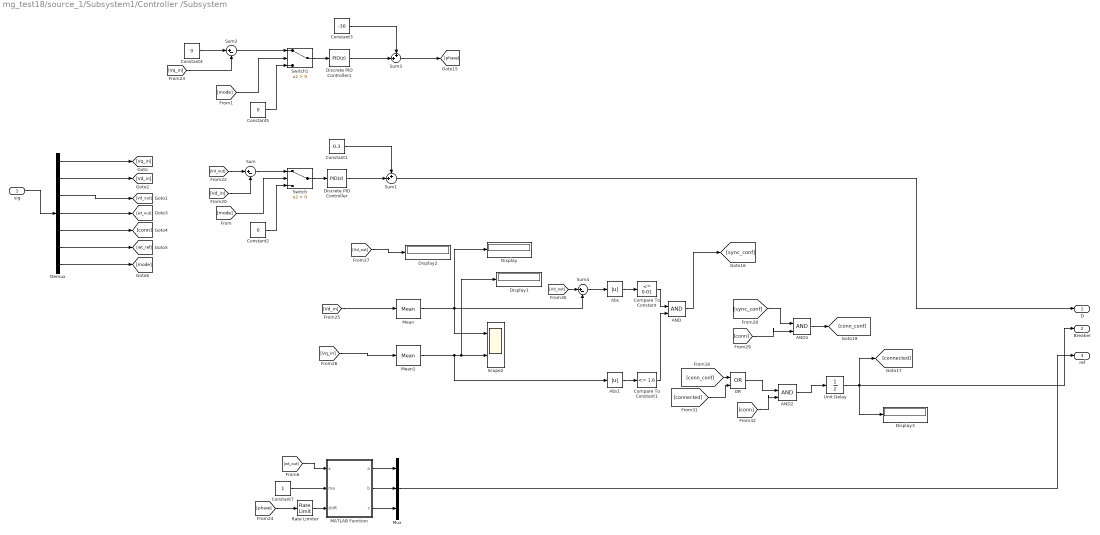
== system mg_test18/source_1/Subsystem1/Controller /Subsystem ==
  sig : Inport
  AND : Logic  IconShape=distinctive  AllPortsSameDT=off  OutDataTypeStr=boolean
  AND1 : Logic  IconShape=distinctive  AllPortsSameDT=off  OutDataTypeStr=boolean
  AND2 : Logic  IconShape=distinctive  AllPortsSameDT=off  OutDataTypeStr=boolean
  Abs : Abs
  Abs1 : Abs
  Compare To Constant : simulink/Logic and Bit Operations/Compare To Constant  relop=<=  const=0.01  OutDataTypeStr=boolean
  Compare To Constant1 : simulink/Logic and Bit Operations/Compare To Constant  relop=<=  const=1.6  OutDataTypeStr=boolean
  Constant1 : Constant  Value=0.3
  Constant2 : Constant  Value=0
  Constant3 : Constant  Value=-30
  Constant4 : Constant  Value=0
  Constant5 : Constant  Value=0
  Constant7 : Constant
  Demux : Demux  Outputs=7
  Discrete PID Controller : simulink/Continuous/PID Controller  Controller=PID  TimeDomain=Discrete-time  SampleTime=Ts_Power  IntegratorMethod=Forward Euler  FilterMethod=Forward Euler  Form=Parallel  UseFilter=on  ControllerParametersSource=internal  P=0.005  I=2  D=0  N=100  InitialConditionSource=internal  InitialConditionForIntegrator=0  InitialConditionForFilter=0  ExternalReset=none  LimitOutput=off  UpperSaturationLimit=inf  LowerSaturationLimit=-inf  LinearizeAsGain=off  AntiWindupMode=none  Kb=1  TrackingMode=off  Kt=1  PParamMin=[]  PParamMax=[]  IParamMin=[]  IParamMax=[]  DParamMin=[]  DParamMax=[]  NParamMin=[]  NParamMax=[]  KbParamMin=[]  KbParamMax=[]  KtParamMin=[]  KtParamMax=[]  POutMin=[]  POutMax=[]  IOutMin=[]  IOutMax=[]  DOutMin=[]  DOutMax=[]  NOutMin=[]  NOutMax=[]  KbOutMin=[]  KbOutMax=[]  KtOutMin=[]  KtOutMax=[]  IntegratorOutMin=[]  IntegratorOutMax=[]  FilterOutMin=[]  FilterOutMax=[]  SumOutMin=[]  SumOutMax=[]  SumI1OutMin=[]  SumI1OutMax=[]  SumI2OutMin=[]  SumI2OutMax=[]  SumI3OutMin=[]  SumI3OutMax=[]  SumDOutMin=[]  SumDOutMax=[]  SaturationOutMin=[]  SaturationOutMax=[]  IntegratorContinuousStateAttributes=''  IntegratorStateMustResolveToSignalObject=off  IntegratorRTWStateStorageClass=Auto  FilterContinuousStateAttributes=''  FilterStateMustResolveToSignalObject=off  FilterRTWStateStorageClass=Auto  DifferentiatorICPrevScaledInput=0  DifferentiatorOutMin=[]  DifferentiatorOutMax=[]  FilterDiffOutCoefMin=[]  FilterDiffOutCoefMax=[]  SumDenOutMin=[]  SumDenOutMax=[]  SumNumOutMin=[]  SumNumOutMax=[]  ReciprocalOutMin=[]  ReciprocalOutMax=[]  DivideOutMin=[]  DivideOutMax=[]  TunerSelectOption=Transfer Function Based (PID Tuner App)
  Discrete PID Controller1 : simulink/Continuous/PID Controller  Controller=PID  TimeDomain=Discrete-time  SampleTime=Ts_Power  IntegratorMethod=Forward Euler  FilterMethod=Forward Euler  Form=Parallel  UseFilter=on  ControllerParametersSource=internal  P=1  I=2  D=0  N=100  InitialConditionSource=internal  InitialConditionForIntegrator=0  InitialConditionForFilter=0  ExternalReset=none  LimitOutput=off  UpperSaturationLimit=inf  LowerSaturationLimit=-inf  LinearizeAsGain=off  AntiWindupMode=none  Kb=1  TrackingMode=off  Kt=1  PParamMin=[]  PParamMax=[]  IParamMin=[]  IParamMax=[]  DParamMin=[]  DParamMax=[]  NParamMin=[]  NParamMax=[]  KbParamMin=[]  KbParamMax=[]  KtParamMin=[]  KtParamMax=[]  POutMin=[]  POutMax=[]  IOutMin=[]  IOutMax=[]  DOutMin=[]  DOutMax=[]  NOutMin=[]  NOutMax=[]  KbOutMin=[]  KbOutMax=[]  KtOutMin=[]  KtOutMax=[]  IntegratorOutMin=[]  IntegratorOutMax=[]  FilterOutMin=[]  FilterOutMax=[]  SumOutMin=[]  SumOutMax=[]  SumI1OutMin=[]  SumI1OutMax=[]  SumI2OutMin=[]  SumI2OutMax=[]  SumI3OutMin=[]  SumI3OutMax=[]  SumDOutMin=[]  SumDOutMax=[]  SaturationOutMin=[]  SaturationOutMax=[]  IntegratorContinuousStateAttributes=''  IntegratorStateMustResolveToSignalObject=off  IntegratorRTWStateStorageClass=Auto  FilterContinuousStateAttributes=''  FilterStateMustResolveToSignalObject=off  FilterRTWStateStorageClass=Auto  DifferentiatorICPrevScaledInput=0  DifferentiatorOutMin=[]  DifferentiatorOutMax=[]  FilterDiffOutCoefMin=[]  FilterDiffOutCoefMax=[]  SumDenOutMin=[]  SumDenOutMax=[]  SumNumOutMin=[]  SumNumOutMax=[]  ReciprocalOutMin=[]  ReciprocalOutMax=[]  DivideOutMin=[]  DivideOutMax=[]  TunerSelectOption=Transfer Function Based (PID Tuner App)
  Display{,1..3} (4 alike) : Display
      Display settings: Decimation=4
      Display1 settings: Decimation=4
      Display2 settings: Decimation=4
  MATLAB Function : MATLAB Function  TreatAsAtomicUnit=on
  Mean : powerlib_meascontrol/Measurements/Mean  Freq=20  Vinit=0  Ts=0
  Mean1 : powerlib_meascontrol/Measurements/Mean  Freq=20  Vinit=5  Ts=0
  Mux : Mux  Inputs=3
  OR : Logic  Operator=OR  IconShape=distinctive  AllPortsSameDT=off  OutDataTypeStr=boolean
  Rate Limiter : RateLimiter  RisingSlewLimit=100  FallingSlewLimit=-100
  Scope2 : Scope  NumInputPorts=2
  Sum : Sum  Inputs=|+-
  Sum1 : Sum  Inputs=++|
  Sum2 : Sum  Inputs=|+-
  Sum3 : Sum  Inputs=++|
  Sum4 : Sum  Inputs=|+-
  Switch : Switch  Criteria=u2 > Threshold
  Switch1 : Switch  Criteria=u2 > Threshold
  Unit Delay : UnitDelay  SampleTime=Ts_Power
  D : Outport
  Breaker : Outport  Port=2
  ref : Outport  Port=3
  wires:
  Rate Limiter/1 -> MATLAB Function/3(shift)
  [Vd_in] -> Mean/1
  Sum1/1 -> D/1
  [Vq_in] -> Sum2/2
  MATLAB Function/3(c) -> Mux/3
  [Vd_out] -> Sum/1
  Mean/1 -> Sum4/2, Scope2/1, Display/1
  MATLAB Function/1(a) -> Mux/1
  Mean1/1 -> Abs1/1, Display1/1, Scope2/2
  Mux/1 -> ref/1
  [wt_out] -> MATLAB Function/1(x)
  Constant3/1 -> Sum3/1
  [connected] -> OR/2
  Sum4/1 -> Abs/1
  Constant4/1 -> Sum2/1
  AND2/1 -> Unit Delay/1
  AND/1 -> [sync_conf]
  Abs/1 -> Compare To Constant/1
  Constant7/1 -> MATLAB Function/2(ma)
  [Vd_in] -> Sum/2
  Sum3/1 -> [phase]
  Constant1/1 -> Sum1/1
  [Vd_out] -> Sum4/1
  [sync_conf] -> AND1/1
  MATLAB Function/2(b) -> Mux/2
  Abs1/1 -> Compare To Constant1/1
  Compare To Constant1/1 -> AND/2
  [Vq_in] -> Mean1/1
  Discrete PID Controller1/1 -> Sum3/2
  [Vd_out] -> Display2/1
  Compare To Constant/1 -> AND/1
  Unit Delay/1 -> Breaker/1, Display3/1, [connected]
  Discrete PID Controller/1 -> Sum1/2
  AND1/1 -> [conn_conf]
  [conn] -> AND1/2
  [conn] -> AND2/2
  [phase] -> Rate Limiter/1
  OR/1 -> AND2/1
  [conn_conf] -> OR/1
  Demux/1 -> [Vq_in]
  Demux/3 -> [Vd_out]
  Demux/2 -> [Vd_in]
  Demux/4 -> [wt_out]
  sig/1 -> Demux/1
  Demux/5 -> [conn]
  Demux/6 -> [wt_ref]
  Demux/7 -> [mode]
  Sum/1 -> Switch/1
  Switch/1 -> Discrete PID Controller/1
  Constant2/1 -> Switch/3
  [mode] -> Switch/2
  [mode] -> Switch1/2
  Constant5/1 -> Switch1/3
  Switch1/1 -> Discrete PID Controller1/1
  Sum2/1 -> Switch1/1

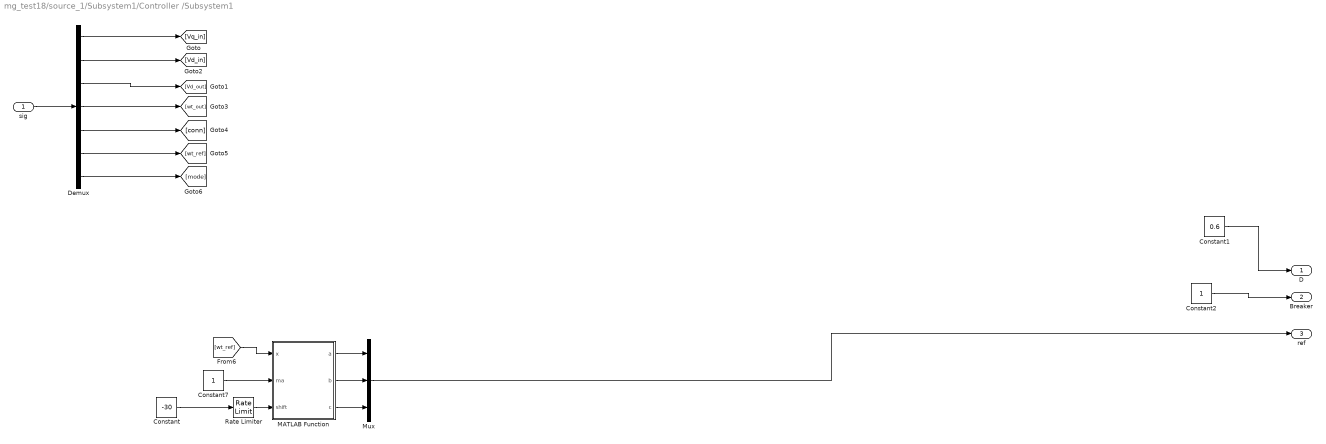
== system mg_test18/source_1/Subsystem1/Controller /Subsystem1 ==
  sig : Inport
  Constant : Constant  Value=-30
  Constant1 : Constant  Value=0.6
  Constant2 : Constant
  Constant7 : Constant
  Demux : Demux  Outputs=7
  MATLAB Function : MATLAB Function  TreatAsAtomicUnit=on
  Mux : Mux  Inputs=3
  Rate Limiter : RateLimiter  RisingSlewLimit=100  FallingSlewLimit=-100
  D : Outport
  Breaker : Outport  Port=2
  ref : Outport  Port=3
  wires:
  Rate Limiter/1 -> MATLAB Function/3(shift)
  MATLAB Function/3(c) -> Mux/3
  MATLAB Function/1(a) -> Mux/1
  Mux/1 -> ref/1
  [wt_ref] -> MATLAB Function/1(x)
  Constant7/1 -> MATLAB Function/2(ma)
  MATLAB Function/2(b) -> Mux/2
  Constant/1 -> Rate Limiter/1
  Constant1/1 -> D/1
  Demux/5 -> [conn]
  sig/1 -> Demux/1
  Demux/2 -> [Vd_in]
  Demux/1 -> [Vq_in]
  Demux/7 -> [mode]
  Demux/4 -> [wt_out]
  Demux/6 -> [wt_ref]
  Demux/3 -> [Vd_out]
  Constant2/1 -> Breaker/1
